simulink model "Tirocinio3Simulink1"  (R2025b)
settings: Solver=VariableStepAuto  StartTime=0.0  StopTime=10.0  RelTol=1e-3
undefined symbols (not defined in the file or in its folder): A_nom, A_real, B_nom, B_real, C_nom, C_real, H_fast, H_kalman, H_slow, M_nom, R_sys, V_fast, V_kalman, V_slow
libraries: simulink x1
settings Model: Creator=Davide  LastModifiedBy=Davide

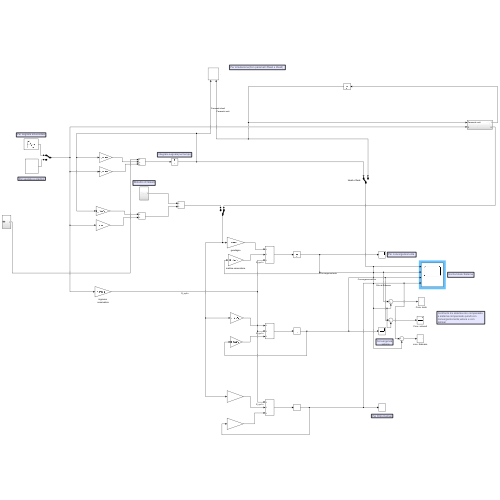
[thumbnail: Simulink's stored preview of the top-level diagram]
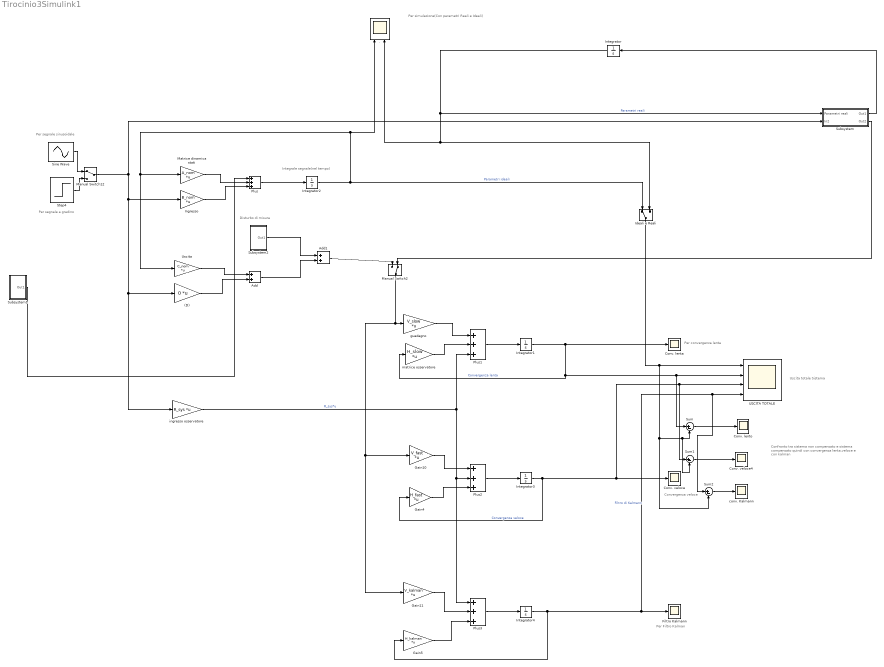
== system Tirocinio3Simulink1 ==
  note: Confronto tra sistema non compensato
      | e sistema compensato quindi con
      | convergenza lenta,veloce e con
      | kalman
  note: Per segnale sinusoidale
  note: Per segnale a gradino
  note: Convergenza
      |        veloce
  note: Per simulazione(Con parametri Reali e Ideali)
  note: Uscita totale Sistema
  note: Disturbo di misura
  note: Per convergenza lenta
  note: Per Filtro Kalman
  note: Integrale segnale(nel tempo)
  (D) : Gain  Gain=0  Multiplication=Matrix(K*u)
  . : Scope  NumInputPorts=2
      settings: ActiveDisplayYMinimum=-8.13487  ActiveDisplayYMaximum=2.00392  DataLoggingVariableName=ScopeData5
  Add : Sum
  Add1 : Sum
  Conv. lenta : Scope
      settings: ActiveDisplayYMinimum=-1.1957781419785687  ActiveDisplayYMaximum=1.2551246240859106
  Conv. lento : Scope
      settings: ActiveDisplayYMinimum=-4131.4771013790105  ActiveDisplayYMaximum=2554.0061024705442  DataLoggingVariableName=ScopeData6
  Conv. veloce : Scope
      settings: ActiveDisplayYMinimum=-442.87907  ActiveDisplayYMaximum=271.15447  DataLoggingVariableName=ScopeData3
  Conv. veloce4 : Scope
      settings: ActiveDisplayYMinimum=-1.73379  ActiveDisplayYMaximum=2.22359  DataLoggingVariableName=ScopeData7
  "Filtro Kalmann " : Scope
      settings: ActiveDisplayYMinimum=-1.82105  ActiveDisplayYMaximum=16.86776  DataLoggingVariableName=ScopeData4
  Gain10 : Gain  Gain=V_fast  Multiplication=Matrix(K*u)
  Gain11 : Gain  Gain=V_kalman  Multiplication=Matrix(K*u)
  Gain4 : Gain  Gain=H_fast  Multiplication=Matrix(K*u)
  Gain5 : Gain  Gain=H_kalman  Multiplication=Matrix(K*u)
  Ideali e Reali : ManualSwitch
  Ingresso : Gain  Gain=B_nom  Multiplication=Matrix(K*u)
  Integrator : Integrator  InitialCondition=[1 -1 0 0]  AbsoluteTolerance=1
  Integrator1 : Integrator  InitialCondition=[0 0 0 0]  AbsoluteTolerance=1
  Integrator2 : Integrator  InitialCondition=[1 -1 0 0]  AbsoluteTolerance=1
  Integrator3 : Integrator  InitialCondition=[0 0 0 0]  AbsoluteTolerance=1
  Integrator4 : Integrator  InitialCondition=[0 0 0 0]  AbsoluteTolerance=1
  Manual Switch12 : ManualSwitch
  Manual Switch2 : ManualSwitch  CurrentSetting=0
  Matrice dinamica stati : Gain  Gain=A_nom  Multiplication=Matrix(K*u)
  Plus{,1..3} (4 alike) : Sum  Inputs=+++
  Sine Wave : Sin  Frequency=4  SampleTime=0
  Step4 : Step  SampleTime=0
  Subsystem : Subsystem
  Subsystem1 : Subsystem
  Subsystem2 : Subsystem
  Sum : Sum  Inputs=|+-
  Sum1 : Sum  Inputs=|+-
  Sum2 : Sum  Inputs=|+-
  USCITA TOTALE : Scope  NumInputPorts=4
      settings: ActiveDisplayString=3  ActiveDisplayYMinimum=-0.51944  ActiveDisplayYMaximum=4.2247  DataLoggingVariableName=ScopeData2
  Uscita : Gain  Gain=C_nom  Multiplication=Matrix(K*u)
  conv. Kalmann : Scope
      settings: ActiveDisplayYMinimum=-1.57205  ActiveDisplayYMaximum=3.84447
  guadagno : Gain  Gain=V_slow  Multiplication=Matrix(K*u)
  ingresso osservatore : Gain  Gain=R_sys  Multiplication=Matrix(K*u)
  matrice osservatore : Gain  Gain=H_slow  Multiplication=Matrix(K*u)
  wires:
  Gain10/1 -> Plus2/1
  Integrator2/1 -> Uscita/1, Matrice dinamica stati/1, ./1, Ideali e Reali/1  "Parametri ideali"
  Integrator3/1 -> USCITA TOTALE/3, Sum1/1, Conv. veloce/1, Gain4/1  "Convergenza veloce"
  Sum2/1 -> conv. Kalmann/1
  Ingresso/1 -> Plus/3
  Integrator/1 -> ./2, Ideali e Reali/2, Subsystem/1(Parametri reali)  "Parametri reali"
  Gain5/1 -> Plus3/3
  Plus/1 -> Integrator2/1
  Add/1 -> Add1/2
  Plus3/1 -> Integrator4/1
  Plus1/1 -> Integrator1/1
  matrice osservatore/1 -> Plus1/2
  Matrice dinamica stati/1 -> Plus/2
  Sum/1 -> Conv. lento/1
  Gain4/1 -> Plus2/3
  Step4/1 -> Manual Switch12/2
  Plus2/1 -> Integrator3/1
  Ideali e Reali/1 -> Sum2/2, Sum1/2, Sum/2, USCITA TOTALE/1
  Gain11/1 -> Plus3/2
  Sum1/1 -> Conv. veloce4/1
  Integrator4/1 -> Gain5/1, "Filtro Kalmann "/1, Sum2/1, USCITA TOTALE/4  "Filtro di Kalmann"
  ingresso osservatore/1 -> Plus1/3, Plus3/1, Plus2/2  "R_sys*u"
  Manual Switch2/1 -> Gain11/1, Gain10/1, guadagno/1
  (D)/1 -> Add/2
  Uscita/1 -> Add/1
  guadagno/1 -> Plus1/1
  Add1/1 -> Manual Switch2/1
  Sine Wave/1 -> Manual Switch12/1
  Integrator1/1 -> matrice osservatore/1, USCITA TOTALE/2, Sum/1, Conv. lenta/1  "Convergenza lenta"
  Manual Switch12/1 -> Subsystem/2(In2), ingresso osservatore/1, (D)/1, Ingresso/1
  Subsystem/1(Out1) -> Integrator/1
  Subsystem/2(Out2) -> Manual Switch2/2
  Subsystem1/1(Out1) -> Plus/1
  Subsystem2/1(Out1) -> Add1/1

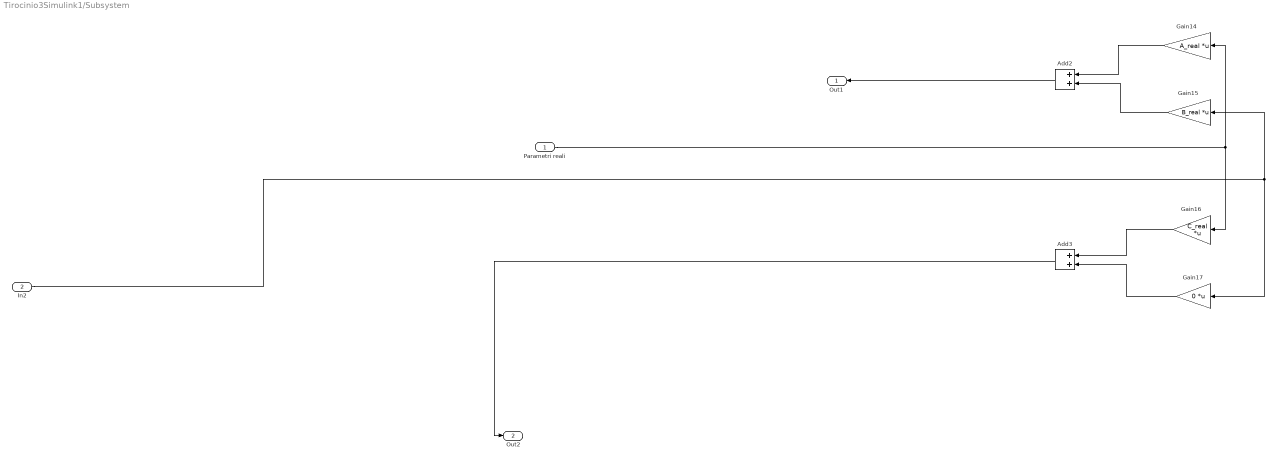
== system Tirocinio3Simulink1/Subsystem ==
  Parametri reali : Inport
  In2 : Inport  Port=2
  Add2 : Sum
  Add3 : Sum
  Gain14 : Gain  Gain=A_real  Multiplication=Matrix(K*u)
  Gain15 : Gain  Gain=B_real  Multiplication=Matrix(K*u)
  Gain16 : Gain  Gain=C_real  Multiplication=Matrix(K*u)
  Gain17 : Gain  Gain=0  Multiplication=Matrix(K*u)
  Out1 : Outport
  Out2 : Outport  Port=2
  wires:
  Gain14/1 -> Add2/1
  Gain16/1 -> Add3/1
  Gain15/1 -> Add2/2
  Add2/1 -> Out1/1
  Parametri reali/1 -> Gain16/1, Gain14/1
  Gain17/1 -> Add3/2
  In2/1 -> Gain17/1, Gain15/1
  Add3/1 -> Out2/1

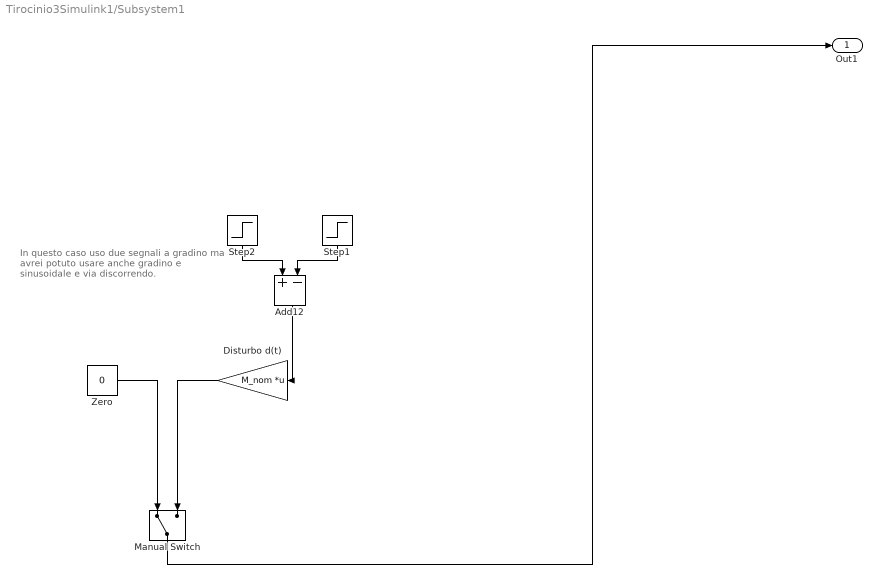
== system Tirocinio3Simulink1/Subsystem1 ==
  note: In questo caso uso due segnali a
      | gradino ma avrei potuto usare
      | anche gradino e sinusoidale e via
      | discorrendo.
  Add12 : Sum  Inputs=+-
  Disturbo d(t) : Gain  Gain=M_nom  Multiplication=Matrix(K*u)
  Manual Switch : ManualSwitch
  Step1 : Step  Time=2  After=4  SampleTime=0
  Step2 : Step  Time=4  After=4  SampleTime=0
  Zero : Constant  Value=0  OutDataTypeStr=Inherit: Inherit via back propagation
  Out1 : Outport
  wires:
  Zero/1 -> Manual Switch/1
  Step1/1 -> Add12/2
  Manual Switch/1 -> Out1/1
  Add12/1 -> Disturbo d(t)/1
  Disturbo d(t)/1 -> Manual Switch/2
  Step2/1 -> Add12/1

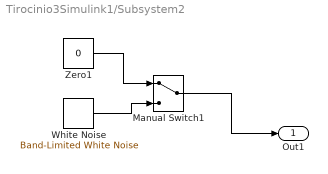
== system Tirocinio3Simulink1/Subsystem2 ==
  Manual Switch1 : ManualSwitch
  White Noise : simulink/Sources/Band-Limited White Noise  Cov=[0.0001]  Ts=0.01  seed=[23341]
  Zero1 : Constant  Value=0  OutDataTypeStr=Inherit: Inherit via back propagation
  Out1 : Outport
  wires:
  White Noise/1 -> Manual Switch1/2
  Zero1/1 -> Manual Switch1/1
  Manual Switch1/1 -> Out1/1
